simulink model "V126_L3_UMS"  (R2020b)
settings: Solver=VariableStepAuto  StartTime=0.0  StopTime=400  MaxStep=0.01  RelTol=1e-3
settings Model: Creator=td  LastModifiedBy=Maxim
settings DataIOCC: ReturnWorkspaceOutputs=off
settings DebuggingCC: ArithmeticOperatorsInVariantConditions=warning
settings SFSimCC: CustomCodeUndefinedFunction=UseInterfaceOnly

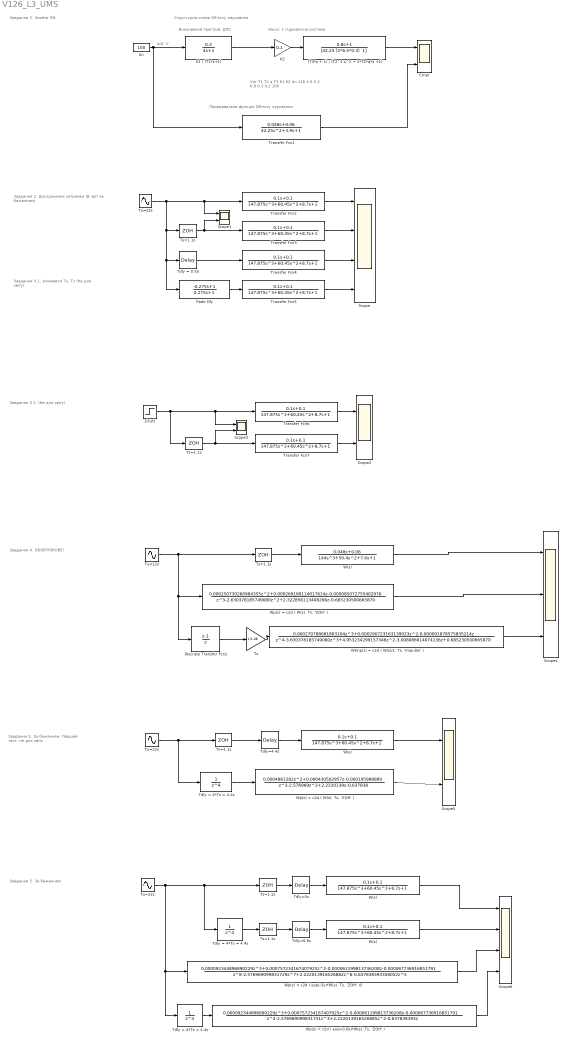
== system V126_L3_UMS ==
  note: Завдання 2.
      | Знайти ПФ
  note: Передавальна функція Об'єкту керування
  note: u(t), V
  note: Насос + гідравлічна система
  note: Виконавчий пристрій, ДПС
  note: Структурна схема Об'єкту керування
  note: Завдання 3.2.
      | (Не для звіту)
  note: Завдання 4.
      | ОБОВ'ЯЗКОВЕ!
  note: Завдання 5.
      | За бажанням
  note: Завдання 5.
      | За бажанням.
      | Перший тест,
      | не для звіту
  note: Завдання 2.
      | Дослідження
      | затримки
      | (В звіт за бажанням)
  note: Завдання 3.1.
      | змінювати Tu, Ts
      | (Не для звіту)
  note: Var	T1	T2	q	T3	K1	K2	Un
      | 126	4	6	0,3	0.8	0.3	0,2	100
  "   Ts=1.1s  " : ZeroOrderHold  SampleTime=1.1
  "   Ts=1.1s   " : ZeroOrderHold  SampleTime=1.1
  "   W(s)   " : TransferFcn  Numerator=[0.1 0.1]  Denominator=[147.875 60.45 8.7 1]
  "  Tdly = 4*Ts = 4.4s " : DiscreteTransferFcn  Denominator="[1  0 0 0 0]"  SampleTime=1.1
  "  Ts=1.1s  " : ZeroOrderHold  SampleTime=1.1
  "  Tu=22s   " : Sin  Frequency=2*pi*(1/11)  SampleTime=0
  "  W(s)  " : TransferFcn  Numerator=[0.1 0.1]  Denominator=[147.875 60.45 8.7 1]
  " Tdly = 4*Ts = 4.4s " : DiscreteTransferFcn  Denominator="[1  0 0 0 0]"  SampleTime=1.1
  " Ts=1.1s  " : ZeroOrderHold  SampleTime=1.08
  " Tu=22s  " : Sin  Frequency=2*pi*(1/11)  SampleTime=0
  " W(s) " : TransferFcn  Numerator=[0.1 0.1]  Denominator=[147.875 60.45 8.7 1]
  (T3*s + 1) / (T2^2 s^2 + 2*T2*q*s +1) : TransferFcn  Numerator=[0.8 1]  Denominator="[42.25 (2*6.5*0.3)  1]"
  1(t-st) : Step  Time=0.1  SampleTime=0
  Cmpr : Scope  NumInputPorts=2
  Discrete Transfer Fcn2 : DiscreteTransferFcn  Numerator=[ 1 -1]  Denominator=[1 0]  SampleTime=1.08
  K1 / (T1*s+1) : TransferFcn  Numerator=[0.3]  Denominator=[4 1]
  K2 : Gain  Gain=0.1
  Pade Dly : TransferFcn  Numerator=[-0.275 1]  Denominator=[0.275 1]
  Scope : Scope  NumInputPorts=4
  Scope{1..3,5} (4 alike) : Scope  NumInputPorts=2
  Scope4 : Scope  NumInputPorts=3
  Scope6 : Scope  NumInputPorts=4
  Tdly = 0.55 : TransportDelay  DelayTime=0.55
  Tdly = 4*Ts = 4.4s : DiscreteTransferFcn  Denominator="[1  0 0 0 0]"  SampleTime=1.1
  Tdly=0.6s : TransportDelay  DelayTime=0.6
  Tdly=4.4s : TransportDelay  DelayTime=4.4
  Tdly=5s : TransportDelay  DelayTime=5
  Transfer Fcn1 : TransferFcn  Numerator=[0.048 0.06]  Denominator=[0 42.25 3.9 1]
  Transfer Fcn{2..7} (6 alike) : TransferFcn  Numerator=[0.1 0.1]  Denominator=[147.875 60.45 8.7 1]
  Ts : Gain  Gain=1/1.08
  Ts=1.1s : ZeroOrderHold  SampleTime=1.1
  "Ts=1.1s " : ZeroOrderHold  SampleTime=1.1
  Tu=22s : Sin  Frequency=2*pi*(1/11)  SampleTime=0
  "Tu=22s  " : Sin  Frequency=2*pi*(1/206)  SampleTime=0
  Un : Constant  Value=100
  W(s) : TransferFcn  Numerator=[0.048 0.06]  Denominator=[144 50.4 7.6 1]
  "Wp(z) = c2d ( W(s), Ts, 'ZOH' )" : DiscreteTransferFcn  Numerator="[0   0.000250730260984355   0.000269188114017614  -0.000085072755402976]"  Denominator="[1  -2.630378185749080   2.322856113408266  -0.685230500665870]"  SampleTime=1.08
  "Wp(z) = c2d ( W(s), Ts, 'ZOH' ) " : DiscreteTransferFcn  Numerator="[0   0.0004861282   0.000430502957  -0.000195988889]"  Denominator="[1  -2.576969   2.2220139  -0.637838]"  SampleTime=1.1
  "Wp(z) = c2d ( exp(-0.6s)*W(s), Ts, 'ZOH' ) " : DiscreteTransferFcn  Numerator="[0.000092344896890229   0.000757234167407925  -0.000061199813736208  -0.000067736916851791]"  Denominator="[1.000  -2.576969099831731   2.222013916526885  -0.637838393 0]"  SampleTime=1.1
  "Wp(z) = c2d ( exp(-5s)*W(s), Ts, 'ZOH' )3" : DiscreteTransferFcn  Numerator="[0.000092344896890229   0.000757234167407925  -0.000061199813736208  -0.000067736916851791]"  Denominator="[1  -2.576969099831729   2.222013916526882  -0.637838393358052 0 0 0 0 0]"  SampleTime=1.1
  "Wtmp(z) = c2d ( W(s)/s, Ts, 'Impulse' )" : DiscreteTransferFcn  Numerator="[0   0.000270788681863104   0.000290723163139023  -0.000091878575835214 0 ]"  Denominator="[1  -3.630378185749080   4.953234299157346  -3.008086614074136   0.685230500665870]"  SampleTime=1.08
  wires:
  Un/1 -> Transfer Fcn1/1, K1 / (T1*s+1)/1
  K1 / (T1*s+1)/1 -> K2/1
  K2/1 -> (T3*s + 1) / (T2^2 s^2 + 2*T2*q*s +1)/1
  (T3*s + 1) / (T2^2 s^2 + 2*T2*q*s +1)/1 -> Cmpr/1
  Transfer Fcn1/1 -> Cmpr/2
  Tu=22s/1 -> Pade Dly/1, Tdly = 0.55/1, Ts=1.1s/1, Transfer Fcn2/1, Scope1/1
  Ts=1.1s/1 -> Transfer Fcn3/1, Scope1/2
  Tdly = 0.55/1 -> Transfer Fcn4/1
  Transfer Fcn2/1 -> Scope/1
  Transfer Fcn3/1 -> Scope/2
  Transfer Fcn4/1 -> Scope/3
  Transfer Fcn5/1 -> Scope/4
  Pade Dly/1 -> Transfer Fcn5/1
  1(t-st)/1 -> "Ts=1.1s "/1, Transfer Fcn6/1, Scope3/1
  Transfer Fcn7/1 -> Scope2/2
  "Ts=1.1s "/1 -> Transfer Fcn7/1, Scope3/2
  Transfer Fcn6/1 -> Scope2/1
  " Ts=1.1s  "/1 -> W(s)/1
  "Tu=22s  "/1 -> Discrete Transfer Fcn2/1, "Wp(z) = c2d ( W(s), Ts, 'ZOH' )"/1, " Ts=1.1s  "/1
  W(s)/1 -> Scope4/1
  "Wp(z) = c2d ( W(s), Ts, 'ZOH' )"/1 -> Scope4/2
  Discrete Transfer Fcn2/1 -> Ts/1
  Ts/1 -> "Wtmp(z) = c2d ( W(s)/s, Ts, 'Impulse' )"/1
  "Wtmp(z) = c2d ( W(s)/s, Ts, 'Impulse' )"/1 -> Scope4/3
  " W(s) "/1 -> Scope5/1
  "Wp(z) = c2d ( W(s), Ts, 'ZOH' ) "/1 -> Scope5/2
  " Tu=22s  "/1 -> Tdly = 4*Ts = 4.4s/1, "  Ts=1.1s  "/1
  Tdly=4.4s/1 -> " W(s) "/1
  "  Ts=1.1s  "/1 -> Tdly=4.4s/1
  Tdly = 4*Ts = 4.4s/1 -> "Wp(z) = c2d ( W(s), Ts, 'ZOH' ) "/1
  " Tdly = 4*Ts = 4.4s "/1 -> "   Ts=1.1s   "/1
  Tdly=5s/1 -> "  W(s)  "/1
  "   Ts=1.1s  "/1 -> Tdly=5s/1
  "   W(s)   "/1 -> Scope6/2
  "  W(s)  "/1 -> Scope6/1
  "   Ts=1.1s   "/1 -> Tdly=0.6s/1
  Tdly=0.6s/1 -> "   W(s)   "/1
  "  Tu=22s   "/1 -> "  Tdly = 4*Ts = 4.4s "/1, "Wp(z) = c2d ( exp(-5s)*W(s), Ts, 'ZOH' )3"/1, " Tdly = 4*Ts = 4.4s "/1, "   Ts=1.1s  "/1
  "Wp(z) = c2d ( exp(-5s)*W(s), Ts, 'ZOH' )3"/1 -> Scope6/3
  "  Tdly = 4*Ts = 4.4s "/1 -> "Wp(z) = c2d ( exp(-0.6s)*W(s), Ts, 'ZOH' ) "/1
  "Wp(z) = c2d ( exp(-0.6s)*W(s), Ts, 'ZOH' ) "/1 -> Scope6/4
